simulink model "px4demo_QGC_tune"  (R2017b)
settings: Solver=FixedStepAuto  StartTime=0.0  StopTime=inf  RelTol=1e-3  EnableMultiTasking=on
InitFcn:
  | %param_define;
  | 
  | SL_MSG = Pixhawk_CSC.Parameter( {int32(1), 'SL_MSG'}  );
  | SL_TEST = Pixhawk_CSC.Parameter( {single(14.7), 'SL_TEST'}  );
libraries: pixhawk_slib_misc_utils x1
Description:
  | This demo model showcases how to use custom storage class parameters to be tunable over QGroundControl.
  | 
  | Note, that you may need to delete the parameters.xml file to properly update the list of parameters. This file is located :
  | C:\px4_firmware_test\Firmware\build_<fimware_variant>\parameters.xml
  | Where <firmware_variant> could be px4fmu-v3_default or px4fmu-v2_default, etc
  | 
  | 
  | Use the 'px4_simulink_app_params.c' file to define the new parameters that will show up in QGC
settings Model: Creator=darenlee  LastModifiedBy=skuznick
settings SolverCC: PositivePriorityOrder=on
settings DataIOCC: LimitDataPoints=on
settings OptimizationCC: DefaultParameterBehavior=Inlined  LifeSpan=1  MaxStackSize=64
settings DebuggingCC: AllowSymbolicDim=off  SFUnexpectedBacktrackingDiag=warning  SFNoUnconditionalDefaultTransitionDiag=warning  SFExecutionAtInitializationDiag=none
settings HardwareCC: ProdBitPerPointer=32  ProdBitPerSizeT=32  ProdBitPerPtrDiffT=32  ProdLargestAtomicInteger=Long  ProdLargestAtomicFloat=Double  ProdWordSize=32  ProdHWDeviceType=ARM Compatible->ARM Cortex
settings ModelReferenceCC: PropagateSignalLabelsOutOfModel=off
settings SFSimCC: MATLABDynamicMemAlloc=off
settings RTWCC: SystemTargetFile=ert.tlc  HardwareBoard=Pixhawk PX4  TemplateMakefile=ert_default_tmf  GenerateReport=on  CustomSource=px4_simulink_app_params.c  Toolchain=Pixhawk Toolchain  IncludeHyperlinkInReport=on  LaunchReport=on  GenerateTraceInfo=on  GenerateTraceReport=on  GenerateTraceReportSl=on  GenerateTraceReportSf=on  GenerateTraceReportEml=on
settings RTWCC: CustomHeaderCode=|
  | #include <px4_config.h>
  | #include <px4_tasks.h>
  | #include <px4_posix.h>
  | #include <unistd.h>
  | #include <stdio.h>
  | #include <poll.h>
  | #include <string.h>
settings CodeAppCC: ForceParamTrailComments=on  IgnoreCustomStorageClasses=off  OperatorAnnotations=on  StateflowObjectComments=on  MATLABSourceComments=on
settings ERTTargetCC: MultiwordLength=2048  ExtModeTransport=1  ExtModeMexFile=ext_serial_win32_comm  ExtModeMexArgs=1 7 115200  InlinedParameterPlacement=NonHierarchical  ERTCustomFileTemplate=px4_codertarget_file_process.tlc  ConvertIfToSwitch=off  SuppressUnreachableDefaultCases=off
settings ConfigComp: CovMetricSettings=dw  CovHtmlReporting=on  CovSaveCumulativeToWorkspaceVar=on  CovSaveSingleToWorkspaceVar=on  CovExternalEMLEnable=off

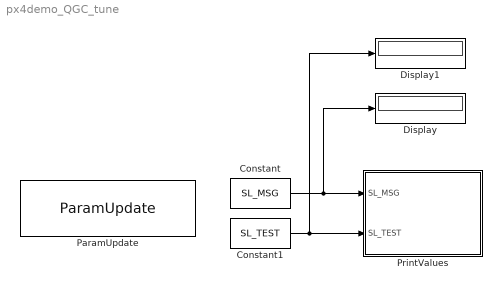
== system px4demo_QGC_tune ==
  Constant : Constant  Value=SL_MSG  SampleTime=-1
  Constant1 : Constant  Value=SL_TEST  SampleTime=-1
  Display : Display
  Display1 : Display
  ParamUpdate : pixhawk_slib_misc_utils/ParamUpdate  Unformatted_StrSet=0  TLC_StrSet=0  NumParams=0  Ts=0
      settings: SourceProductName=Pixhawk Target Blocks
  PrintValues : MATLAB Function  TreatAsAtomicUnit=on
  wires:
  Constant/1 -> Display/1, PrintValues/1(SL_MSG)
  Constant1/1 -> Display1/1, PrintValues/2(SL_TEST)

== matlab function px4demo_QGC_tune/PrintValues ==
  data: SL_MSG input; SL_TEST input
function print_fcn(SL_MSG,SL_TEST)
if coder.target('rtw')
msg_str = coder.const(['SL_MSG = %d SL_TEST = %8.4f',uint8(10),uint8(0)]);
coder.ceval('PX4_INFO',coder.rref(msg_str),SL_MSG,SL_TEST);
end
end
